simulink subsystem "PieroControlado_1mZ"  (R2023b)
settings: Solver=VariableStepAuto  StartTime=0.0  StopTime=10.0  RelTol=1e-3
undefined symbols (not defined in the file): DiscIntNeverNeededParam
settings Model: Creator=Carlos  LastModifiedBy=Carlos

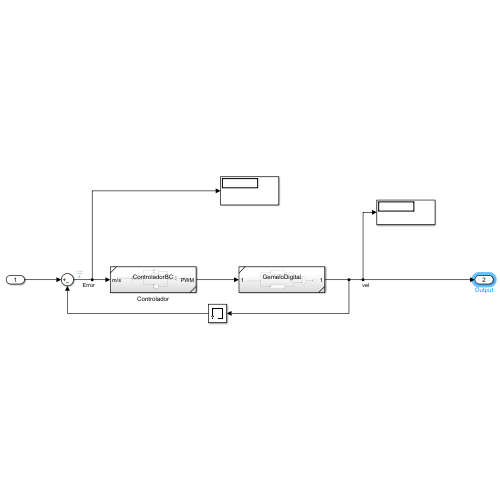
[thumbnail: Simulink's stored preview of the top-level diagram]
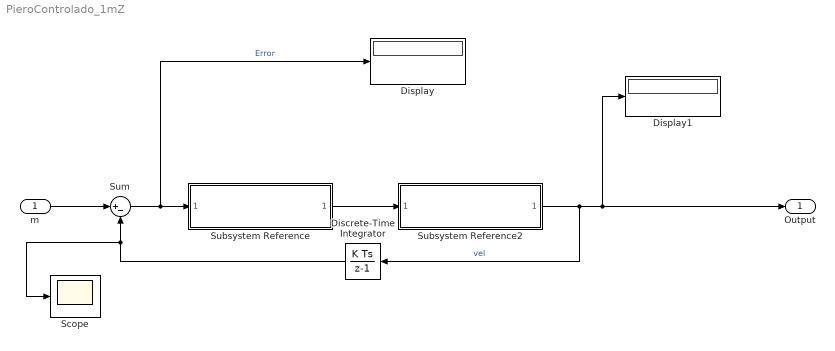
== system PieroControlado_1mZ ==
  m : Inport  OutDataTypeStr=double
  Discrete-Time Integrator : DiscreteIntegrator  SampleTime=-1  ICPrevOutput=DiscIntNeverNeededParam  ICPrevScaledInput=DiscIntNeverNeededParam
  Display : Display
  Display1 : Display
  Scope : Scope
  Subsystem Reference : Subsystem  ReferencedSubsystem=ControladorPos1mZ
  Subsystem Reference2 : Subsystem  ReferencedSubsystem=GemeloDigitalZ
  Sum : Sum  Inputs=|+-
  Output : Outport  OutDataTypeStr=double
  wires:
  Sum/1 -> Display/1, Subsystem Reference/1  "Error"
  Subsystem Reference2/1 -> Output/1, Display1/1, Discrete-Time Integrator/1  "vel"
  Subsystem Reference/1 -> Subsystem Reference2/1
  m/1 -> Sum/1
  Discrete-Time Integrator/1 -> Sum/2, Scope/1
